simulink model "LQR_Integrate_model"  (R2015a)
settings: Solver=ode45  StartTime=0.0  StopTime=30  RelTol=1e-3
values from neighbouring files (symbols this model uses):
  dSamplingPeriod = 0.01    [LQR_Integrate_config.m]    (also in PFC_Integrate_config.m; PFC_config.m)
  gain_lqr_f = gain_lqr_buff(:,1:4)    [LQR_Integrate_config.m]
  gain_lqr_g = -gain_lqr_buff(:,5:6)    [LQR_Integrate_config.m]
  plant = ss( Ac, Bc, Cc, Dc )    [LQR_Integrate_config.m]    (also in PFC_Integrate_config.m; PFC_config.m)
undefined symbols (not defined in the file or in its folder): sigbuilder_block
libraries: simulink x3
settings Model: Creator=hamada  LastModifiedBy=hamada

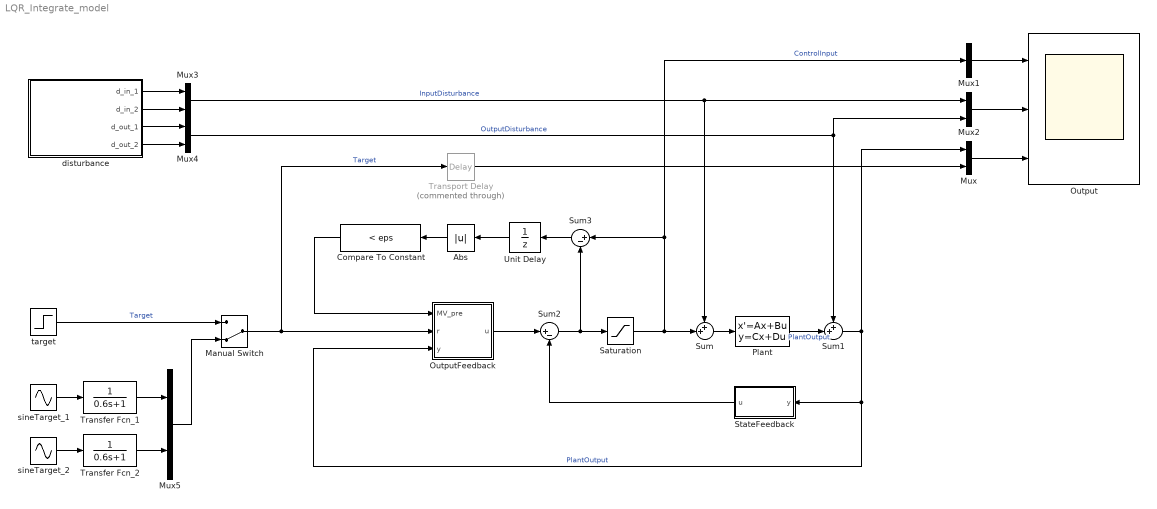
== system LQR_Integrate_model ==
  Abs : Abs
  Compare To Constant : simulink/Logic and Bit Operations/Compare To Constant  relop=<  const=eps  OutDataTypeStr=boolean
  Manual Switch : ManualSwitch  CurrentSetting=0
  Mux{,2..5} (5 alike) : Mux  Inputs=2
  Mux1 : Mux  Inputs=1
  Output : Scope  NumInputPorts=3
      settings: ShowLegends=on  TimeRange=30  YMin=-3~-0.3~-2  YMax=3~0.5~2.5
  OutputFeedback : Subsystem
  Plant : StateSpace  A=plant.a  B=plant.b  C=plant.c  D=plant.d  X0=0
  Saturation : Saturate  UpperLimit=3  LowerLimit=-3
  StateFeedback : Subsystem
  Sum : Sum  Inputs=++|
  Sum1 : Sum  Inputs=++|
  Sum2 : Sum  Inputs=|+-
  Sum3 : Sum  Inputs=|+-
  Transfer Fcn_1 : TransferFcn  Denominator=[0.6 1]
  Transfer Fcn_2 : TransferFcn  Denominator=[0.6 1]
  Transport Delay : TransportDelay  Commented=through  DelayTime=0.45
  Unit Delay : UnitDelay  SampleTime=dSamplingPeriod
  disturbance : Subsystem  Tag=STV Subsys  LoadFcn=sigbuilder_block('load');  StartFcn=sigbuilder_block('start');  StopFcn=sigbuilder_block('stop');  ClipboardFcn=sigbuilder_block('clipboard');  mask(Sigbuilder block){}
      mask help: Simulink:masks:SigbuilderBlock_MD
      mask init:
      | if ~strcmp(get_param(bdroot(gcbh),'SimulationStatus'),'stopped') tuvar = sigbuilder_block('maskInit'); end
      settings: CopyFcn=sigbuilder_block('copy');  DeleteFcn=sigbuilder_block('delete');  ModelCloseFcn=sigbuilder_block('modelClose');  PreSaveFcn=sigbuilder_block('preSave');  PauseFcn=sigbuilder_block('pause');  ContinueFcn=sigbuilder_block('continue');  NameChangeFcn=sigbuilder_block('namechange');  OpenFcn=sigbuilder_block('open',[437.6 199.2 550.4 400 ]);  CloseFcn=sigbuilder_block('close');
      mask Display: plot(0, 0, 100, 100,[2, 2, 32, 32, 2], [68, 8, 8, 68, 68],[32, 2], [38, 38], [32, 19, 2],[53, 60, 44], [32, 17, 17, 2],[16, 16, 31, 31]);txt = getActiveGroup(gcbh);text(2, 100, txt,'verticalAlignment', 'top');
  sineTarget_1 : Sin  Frequency=2*pi*0.2  SampleTime=0
  sineTarget_2 : Sin  Amplitude=2  Frequency=2*pi*0.1  Phase=-pi/4  SampleTime=0
  target : Step  Time=[1;5]  Before=[0;0]  After=[1;2]  SampleTime=0
  wires:
  Sum2/1 -> Saturation/1, Sum3/2
  Sum1/1 -> OutputFeedback/3(y), StateFeedback/1(y), Mux/1  "PlantOutput"
  Sum/1 -> Plant/1
  Mux3/1 -> Mux2/1, Sum/1  "InputDisturbance"
  Mux/1 -> Output/3
  Mux1/1 -> Output/1
  Mux2/1 -> Output/2
  Plant/1 -> Sum1/2  "PlantOutput"
  disturbance/2(d_in_2) -> Mux3/2
  disturbance/1(d_in_1) -> Mux3/1
  disturbance/4(d_out_2) -> Mux4/2
  disturbance/3(d_out_1) -> Mux4/1
  Mux4/1 -> Mux2/2, Sum1/1  "OutputDisturbance"
  sineTarget_1/1 -> Transfer Fcn_1/1
  sineTarget_2/1 -> Transfer Fcn_2/1
  Transfer Fcn_1/1 -> Mux5/1
  Transfer Fcn_2/1 -> Mux5/2
  target/1 -> Manual Switch/1  "Target"
  Mux5/1 -> Manual Switch/2
  Manual Switch/1 -> Transport Delay/1, OutputFeedback/2(r)  "Target"
  Saturation/1 -> Mux1/1, Sum3/1, Sum/2  "ControlInput"
  StateFeedback/1(u) -> Sum2/2
  OutputFeedback/1(u) -> Sum2/1
  Compare To Constant/1 -> OutputFeedback/1(MV_pre)
  Sum3/1 -> Unit Delay/1
  Abs/1 -> Compare To Constant/1
  Unit Delay/1 -> Abs/1
  Transport Delay/1 -> Mux/2

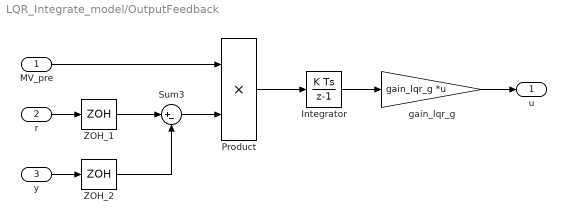
== system LQR_Integrate_model/OutputFeedback ==
  MV_pre : Inport
  r : Inport  Port=2
  y : Inport  Port=3
  Integrator : DiscreteIntegrator  InitialConditionSetting=State (most efficient)  SampleTime=dSamplingPeriod
  Product : Product
  Sum3 : Sum  Inputs=|+-
  ZOH_1 : ZeroOrderHold  SampleTime=dSamplingPeriod
  ZOH_2 : ZeroOrderHold  SampleTime=dSamplingPeriod
  gain_lqr_g : Gain  Gain=gain_lqr_g  Multiplication=Matrix(K*u)
  u : Outport
  wires:
  ZOH_2/1 -> Sum3/2
  y/1 -> ZOH_2/1
  gain_lqr_g/1 -> u/1
  r/1 -> ZOH_1/1
  Product/1 -> Integrator/1
  ZOH_1/1 -> Sum3/1
  Integrator/1 -> gain_lqr_g/1
  Sum3/1 -> Product/2
  MV_pre/1 -> Product/1

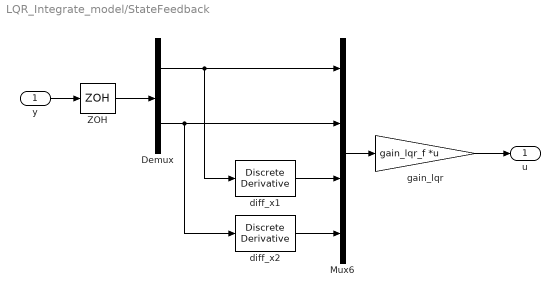
== system LQR_Integrate_model/StateFeedback ==
  y : Inport
  Demux : Demux  Outputs=2
  Mux6 : Mux
  ZOH : ZeroOrderHold  SampleTime=dSamplingPeriod
  diff_x1 : simulink/Discrete/Discrete Derivative  gainval=1.0  ICPrevScaledInput=0.0  InputProcessing=Inherited  OutMin=[]  OutMax=[]  OutDataType=fixdt(1, 16)  OutScaling=2^-10  DoSatur=off
  diff_x2 : simulink/Discrete/Discrete Derivative  gainval=1.0  ICPrevScaledInput=0.0  InputProcessing=Inherited  OutMin=[]  OutMax=[]  OutDataType=fixdt(1, 16)  OutScaling=2^-10  DoSatur=off
  gain_lqr : Gain  Gain=gain_lqr_f  Multiplication=Matrix(K*u)
  u : Outport
  wires:
  Demux/2 -> diff_x2/1, Mux6/2
  Mux6/1 -> gain_lqr/1
  Demux/1 -> Mux6/1, diff_x1/1
  diff_x1/1 -> Mux6/3
  y/1 -> ZOH/1
  diff_x2/1 -> Mux6/4
  ZOH/1 -> Demux/1
  gain_lqr/1 -> u/1

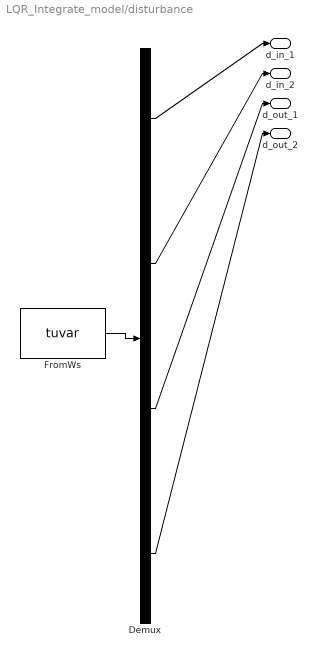
== system LQR_Integrate_model/disturbance ==
  Demux : Demux  Tag=STV Demux
  FromWs : FromWorkspace  Tag=STV FromWs  VariableName=tuvar  SampleTime=0
      SigBuilderData=|
      | common.afterFinalStr = 'Extrapolate'
      | common.sampleTime = 0
      | dataSet(1).timeRange = [0 30]
      | dataSet(1).name = 'Group 1'
      | dataSet(2).timeRange = [0 30]
      | dataSet(2).name = 'Group 2'
      | sbobj.Groups(1).Name = 'Group 1'
      | sbobj.Groups(1).Signals(1).Name = 'd_in_1'
      | sbobj.Groups(1).Signals(1).XData = [0 10 10 30]
      | sbobj.Groups(1).Signals(1).YData = [0 0 0.5 0.5]
      | sbobj.Groups(1).Signals(2).Name = 'd_in_2'
      | sbobj.Groups(1).Signals(2).XData = [0 15 15 30]
      | sbobj.Groups(1).Signals(2).YData = [0 0 -0.25 -0.25]
      | sbobj.Groups(1).Signals(3).Name = 'd_out_1'
      | sbobj.Groups(1).Signals(3).XData = [0 20 20 30]
      | sbobj.Groups(1).Signals(3).YData = [0 0 -0.2 -0.2]
      | sbobj.Groups(1).Signals(4).Name = 'd_out_2'
      | sbobj.Groups(1).Signals(4).XData = [0 25 25 30]
      | sbobj.Groups(1).Signals(4).YData = [0 0 0.4 0.4]
      | sbobj.Groups(1).TimeRange = [0 30]
      | sbobj.Groups(2).Name = 'Group 2'
      | sbobj.Groups(2).Signals(1).Name = 'd_in_1'
      | sbobj.Groups(2).Signals(1).XData = [0 10 10 12.5 12.5 30]
      | sbobj.Groups(2).Signals(1).YData = [0 0 0.2 0.2 0 0]
      | sbobj.Groups(2).Signals(2).Name = 'd_in_2'
      | sbobj.Groups(2).Signals(2).XData = [0 15 15 17.5 17.5 30]
      | sbobj.Groups(2).Signals(2).YData = [0 0 -0.4 -0.4 0 0]
      | sbobj.Groups(2).Signals(3).Name = 'd_out_1'
      | sbobj.Groups(2).Signals(3).XData = [0 20 20 22.5 22.5 30]
      | sbobj.Groups(2).Signals(3).YData = [0 0 2 2 0 0]
      | sbobj.Groups(2).Signals(4).Name = 'd_out_2'
      | sbobj.Groups(2).Signals(4).XData = [0 25 25 27.5 27.5 30]
      | sbobj.Groups(2).Signals(4).YData = [0 0 -1 -1 0 0]
      | sbobj.Groups(2).TimeRange = [0 30]
  d_in_1 : Outport  Tag=STV Outport
  d_in_2 : Outport  Tag=STV Outport  Port=2
  d_out_1 : Outport  Tag=STV Outport  Port=3
  d_out_2 : Outport  Tag=STV Outport  Port=4
  wires:
  FromWs/1 -> Demux/1
  Demux/1 -> d_in_1/1
  Demux/2 -> d_in_2/1
  Demux/3 -> d_out_1/1
  Demux/4 -> d_out_2/1
